simulink model "SimulacionRM20"  (R2020a)
settings: Solver=VariableStepAuto  StartTime=0.0  StopTime=inf  RelTol=1e-3
undefined symbols (not defined in the file): DiscIntNeverNeededParam, Standard_Devices, UDP_Protocol
libraries: sldrtlib x2
settings Model: Creator=alrer  LastModifiedBy=alrer

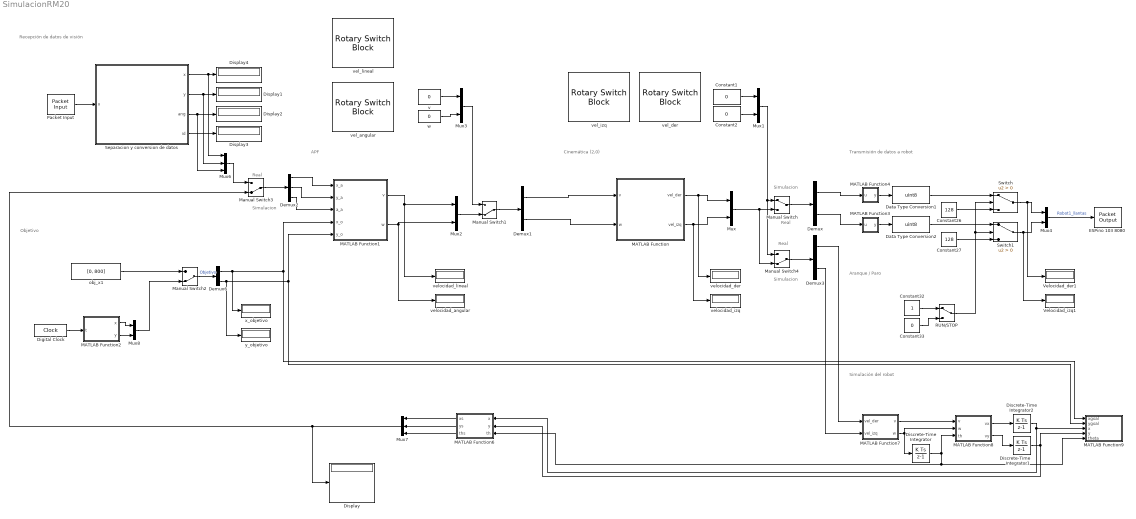
== system SimulacionRM20 ==
  note: Real
  note: Cinemática (2,0)
  note: Transmisión de datos a robot
  note: Aranque / Paro
  note: APF
  note: Objetivo
  note: Recepción de datos de visión
  note: Simulacion
  note: Simulación del robot
  note: Real
  note: Real
  note: Simulacion
  note: Simulacion
  Constant1 : Constant  Value=0
  Constant2 : Constant  Value=0
  Constant26 : Constant  Value=128
  Constant27 : Constant  Value=128
  Constant32 : Constant
  Constant33 : Constant  Value=0
  Data Type Conversion1 : DataTypeConversion  OutMin=0  OutMax=255  OutDataTypeStr=uint8
  Data Type Conversion2 : DataTypeConversion  OutMin=0  OutMax=255  OutDataTypeStr=uint8
  Demux{,1,3,6} (4 alike) : Demux  Outputs=2
  Demux2 : Demux  Outputs=3
  Digital Clock : DigitalClock  SampleTime=-1
  Discrete-Time Integrator : DiscreteIntegrator  SampleTime=-1  ICPrevOutput=DiscIntNeverNeededParam  ICPrevScaledInput=DiscIntNeverNeededParam
  Discrete-Time Integrator1 : DiscreteIntegrator  SampleTime=-1  ICPrevOutput=DiscIntNeverNeededParam  ICPrevScaledInput=DiscIntNeverNeededParam
  Discrete-Time Integrator2 : DiscreteIntegrator  SampleTime=-1  ICPrevOutput=DiscIntNeverNeededParam  ICPrevScaledInput=DiscIntNeverNeededParam
  Display{,1..4} (5 alike) : Display
  ESPino 103 8080 : sldrtlib/Packet Output  SampleTime=0.01  MaxMissedTicks=inf  ShowMissedTicks=off  YieldWhenWaiting=off  DrvName=Standard_Devices/UDP_Protocol  DrvAddress=12001  DrvOptions=[0 8080 49 57 50 46 49 54 56 46 49 51 55 46 49 55 49 0 0 0 0 0 0 0 0 0 0 0 0 0 0 0 0 0 0 0 0 0 0 0 0 0 0 0 0 0 0 0 0 0 0 0 0 0 0 0 0 0 0 0 0 0 0 0 0 0 0 0 0 0 0 0 0 0 0 0 0 0 0 0 0 0 0 0 0 0 0 0 0 0 0 0 0 0 0 0 0 0 0 0 0 0 0 0 0 0 0 0 0 0 0 0 0 0 0 0 0 0 0 0 0 0 0 0 0 0 0 0 0 0 0 0 0 0 0 0 0 0 0 0 0 0 0 0 0 0 0 0 0 0 0 0 0 0 0 0 0 0 0 0 0 0 0 0 0 0 0 0 0 0 0 0 0 0 0 0 0 0 0 0 0 0 0 0 0 0 0 0 0 0 0 0 0 0 0 0 0 0 0 0 0 0 0 0 0 0 0 0 0 0 0 0 0 0 0 0 0 0 0 0 0 0 0 0 0 0 0 0 0 0 0 0 0 0 0 0 0 0 0 0 0 0 0 0 0 0 0 0 0 0 0 0 0 0 0 0]  PacketSize=2  DataTypes='2*uint8'  ShowReady=off  ShowError=off  PacketID=1  ByteOrder=1  InitialValue=[]  FinalValue=[]
      settings: AttributesFormatString=UDP Protocol [12001]
  MATLAB Function : MATLAB Function  TreatAsAtomicUnit=on
  MATLAB Function1 : MATLAB Function  TreatAsAtomicUnit=on
  MATLAB Function2 : MATLAB Function  TreatAsAtomicUnit=on
  MATLAB Function3 : MATLAB Function  TreatAsAtomicUnit=on
  MATLAB Function4 : MATLAB Function  TreatAsAtomicUnit=on
  MATLAB Function6 : MATLAB Function  TreatAsAtomicUnit=on
  MATLAB Function7 : MATLAB Function  TreatAsAtomicUnit=on
  MATLAB Function8 : MATLAB Function  TreatAsAtomicUnit=on
  MATLAB Function9 : MATLAB Function  TreatAsAtomicUnit=on
  Manual Switch : ManualSwitch
  Manual Switch{1..4} (4 alike) : ManualSwitch  CurrentSetting=0
  Mux{,1..4,8} (6 alike) : Mux  Inputs=2
  Mux6 : Mux  Inputs=3
  Mux7 : Mux  Inputs=3
  Packet Input : sldrtlib/Packet Input  SampleTime=0.001  MaxMissedTicks=inf  ShowMissedTicks=off  YieldWhenWaiting=off  DrvName=Standard_Devices/UDP_Protocol  DrvAddress=58624  DrvOptions=[0 58624 49 50 55 46 48 46 48 46 49 0 0 0 0 0 0 0 0 0 0 0 0 0 0 0 0 0 0 0 0 0 0 0 0 0 0 0 0 0 0 0 0 0 0 0 0 0 0 0 0 0 0 0 0 0 0 0 0 0 0 0 0 0 0 0 0 0 0 0 0 0 0 0 0 0 0 0 0 0 0 0 0 0 0 0 0 0 0 0 0 0 0 0 0 0 0 0 0 0 0 0 0 0 0 0 0 0 0 0 0 0 0 0 0 0 0 0 0 0 0 0 0 0 0 0 0 0 0 0 0 0 0 0 0 0 0 0 0 0 0 0 0 0 0 0 0 0 0 0 0 0 0 0 0 0 0 0 0 0 0 0 0 0 0 0 0 0 0 0 0 0 0 0 0 0 0 0 0 0 0 0 0 0 0 0 0 0 0 0 0 0 0 0 0 0 0 0 0 0 0 0 0 0 0 0 0 0 0 0 0 0 0 0 0 0 0 0 0 0 0 0 0 0 0 0 0 0 0 0 0 0 0 0 0 0 0 0 0 0 0 0 0 0 0 0 0 0 0 0 0 0 0 0 0 0]  PacketSize=34  DataTypes='34*int8'  ShowReady=off  ShowError=off  PacketID=1  ByteOrder=1  ShowTimestamp=off
      settings: AttributesFormatString=UDP Protocol [58624]
  RUN/STOP : ManualSwitch
  Separacion y conversion de datos : MATLAB Function  TreatAsAtomicUnit=on
  Switch : Switch  Criteria=u2 > Threshold
  Switch1 : Switch  Criteria=u2 > Threshold
  "Velocidad_der1 " : Display
  Velocidad_izq1 : Display
  obj_x1 : Constant  Value=[0, 800]
  v : Constant  Value=0
  vel_angular : RotarySwitchBlock
      settings: Values={{'-100', '-50', '0', '50', '100'}, [-100 -50 0 50 100]}
  vel_der : RotarySwitchBlock
      settings: Values={{'-400', '-200', '0', '200', '400'}, [-400 -200 0 200 400]}
  vel_izq : RotarySwitchBlock
      settings: Values={{'-400', '-200', '0', '200', '400'}, [-400 -200 0 200 400]}
  vel_lineal : RotarySwitchBlock
      settings: Values={{'-20', '-10', '0', '10', '20'}, [-20000 -10000 0 10000 20000]}
  velocidad_angular : Display
  velocidad_der : Display
  velocidad_izq : Display
  velocidad_lineal : Display
  w : Constant  Value=0
  x_objetivo : Display
  y_objetivo : Display
  wires:
  Packet Input/1 -> Separacion y conversion de datos/1(u)
  Separacion y conversion de datos/1(x) -> Mux6/1, Display4/1
  Separacion y conversion de datos/2(y) -> Display1/1, Mux6/2
  Separacion y conversion de datos/3(ang) -> Display2/1, Mux6/3
  Separacion y conversion de datos/4(id) -> Display3/1
  Switch1/1 -> Velocidad_izq1/1, Mux4/2
  Constant26/1 -> Switch/3
  Switch/1 -> "Velocidad_der1 "/1, Mux4/1
  Constant27/1 -> Switch1/3
  Mux4/1 -> ESPino 103 8080/1  "Robot1_llantas"
  Constant32/1 -> RUN/STOP/1
  Constant33/1 -> RUN/STOP/2
  RUN/STOP/1 -> Switch/2, Switch1/2
  MATLAB Function1/1(v) -> velocidad_lineal/1, Mux2/1
  MATLAB Function1/2(w) -> Mux2/2, velocidad_angular/1
  Manual Switch2/1 -> Demux6/1  "Objetivo"
  Digital Clock/1 -> MATLAB Function2/1(t)
  MATLAB Function2/1(x) -> Mux8/1
  MATLAB Function2/2(y) -> Mux8/2
  Mux8/1 -> Manual Switch2/2
  Demux6/1 -> x_objetivo/1, MATLAB Function9/1(xgoal), MATLAB Function1/4(x_o)
  Demux6/2 -> y_objetivo/1, MATLAB Function9/2(ygoal), MATLAB Function1/5(y_o)
  MATLAB Function/1(vel_der) -> velocidad_der/1, Mux/1
  MATLAB Function/2(vel_izq) -> velocidad_izq/1, Mux/2
  Mux/1 -> Manual Switch4/2, Manual Switch/2
  Manual Switch/1 -> Demux/1
  Demux/2 -> MATLAB Function3/1(u)
  Demux/1 -> MATLAB Function4/1(u)
  Constant2/1 -> Mux1/2
  Constant1/1 -> Mux1/1
  Mux1/1 -> Manual Switch4/1, Manual Switch/1
  Manual Switch1/1 -> Demux1/1
  Mux2/1 -> Manual Switch1/2
  Demux1/1 -> MATLAB Function/1(v)
  Demux1/2 -> MATLAB Function/2(w)
  w/1 -> Mux3/2
  Mux3/1 -> Manual Switch1/1
  MATLAB Function3/1(y) -> Data Type Conversion2/1
  v/1 -> Mux3/1
  MATLAB Function4/1(y) -> Data Type Conversion1/1
  Data Type Conversion1/1 -> Switch/1
  Data Type Conversion2/1 -> Switch1/1
  Mux6/1 -> Manual Switch3/1
  Manual Switch3/1 -> Demux2/1
  Demux2/1 -> MATLAB Function1/1(x_a)
  Demux2/2 -> MATLAB Function1/2(y_a)
  Demux2/3 -> MATLAB Function1/3(a_a)
  MATLAB Function6/1(xs) -> Mux7/1
  Mux7/1 -> Display/1, Manual Switch3/2
  MATLAB Function7/2(w) -> Discrete-Time Integrator/1, MATLAB Function8/2(w)
  MATLAB Function7/1(v) -> MATLAB Function8/1(v)
  Discrete-Time Integrator/1 -> MATLAB Function9/5(theta), MATLAB Function6/3(th), MATLAB Function8/3(th)
  MATLAB Function8/1(vx) -> Discrete-Time Integrator2/1
  MATLAB Function8/2(vy) -> Discrete-Time Integrator1/1
  Discrete-Time Integrator2/1 -> MATLAB Function6/1(x), MATLAB Function9/3(x)
  Discrete-Time Integrator1/1 -> MATLAB Function6/2(y), MATLAB Function9/4(y)
  MATLAB Function6/2(ys) -> Mux7/2
  MATLAB Function6/3(ths) -> Mux7/3
  obj_x1/1 -> Manual Switch2/1
  Manual Switch4/1 -> Demux3/1
  Demux3/2 -> MATLAB Function7/2(vel_izq)
  Demux3/1 -> MATLAB Function7/1(vel_der)

== matlab function SimulacionRM20/MATLAB Function7 ==
  data: vel_der input; v output; vel_izq input; w output
function [v, w] = fcn(vel_der, vel_izq)

    % Parametros Robot
    r = 60;               % Radio de las llantas [mm]
    b = 85;               % Distancia del eje de desplazamiento del robot al centro de las llantas [mm]
    d = 60;               % Distancia del eje de las llantas al punto de control en la dirección de desplazamiento [mm]


    v = (r*vel_der)/2 + (r*vel_izq)/2;
    w = (r*vel_der - r*vel_izq)/(2*b);
end

== matlab function SimulacionRM20/MATLAB Function2 ==
  data: x output; t input; y output
function [x,y] = trayectoria(t)

    % Trayectoria para robot real
    %x = 300*cos(t/10)+600;
    %y = 300*sin(t/10)+450;
    
    % Trayectoria para simulacion (circunferencia)
    %x = 500*cos(30*t);
    %y = 500*sin(30*t);
    
    % Trayectoria para simulacion (lissajous)
    x = 500*sin(30*(t-pi/4));
    y = 500*cos(60*(t-pi/4) + pi/2);
    
end

== matlab function SimulacionRM20/MATLAB Function8 ==
  data: v input; vx output; w input; th input; vy output
function [vx, vy] = fcn(v, w, th)
    
    % Parametros Robot
    r = 60;               % Radio de las llantas [mm]
    b = 85;               % Distancia del eje de desplazamiento del robot al centro de las llantas [mm]
    d = 60;               % Distancia del eje de las llantas al punto de control en la dirección de desplazamiento [mm]

    vx = cos(th)*v - d*sin(th)*w;
    vy = sin(th)*v + d*cos(th)*w;

end

== matlab function SimulacionRM20/MATLAB Function9 ==
  data: xgoal input; ygoal input; x input; y input; theta input
function fcn(xgoal, ygoal, x, y, theta)
    
    % Parametros Robot
    r = 60;               % Radio de las llantas [mm]
    b = 85;               % Distancia del eje de desplazamiento del robot al centro de las llantas [mm]
    d = 60;               % Distancia del eje de las llantas al punto de control en la dirección de desplazamiento [mm]

    % Límites para la visualización de la figura
    xmin=-1000;
    xmax=1000;
    ymin=-1000;
    ymax=1000;
    
    % Dimensiones del robot
    largo_rob=160;
    ancho_rob=160;
    ancho_rueda=15;
    largo_rueda=60;
    
    hold on
    g = findobj('Marker','*');
    set(g,'Visible','off')
    plot(xgoal,ygoal,'*r','MarkerSize',6); % Marca objetivo
    plot(x,y,'.b','MarkerSize',1) % Trazar trayectoria del robot (posición)
    axis([xmin xmax ymin ymax])
    axis square
    grid on
    
    % Cuerpo
    v1=[largo_rob/2;ancho_rob/2];
    v2=[-largo_rob/2;ancho_rob/2];
    v3=[-largo_rob/2;-ancho_rob/2];
    v4=[largo_rob/2;-ancho_rob/2];
    % Llanta derecha
    v5=[-d+largo_rueda/2;b+ancho_rueda/2];
    v6=[-d-largo_rueda/2;b+ancho_rueda/2];
    v7=[-d-largo_rueda/2;b-ancho_rueda/2];
    v8=[-d+largo_rueda/2;b-ancho_rueda/2];
    % Llanta izquierda
    v9=[-d+largo_rueda/2;-b+ancho_rueda/2];
    v10=[-d-largo_rueda/2;-b+ancho_rueda/2];
    v11=[-d-largo_rueda/2;-b-ancho_rueda/2];
    v12=[-d+largo_rueda/2;-b-ancho_rueda/2];
    % Eje entre llantas
    v13=[-d;b];
    v14=[-d;-b];
    %	Rueda frontal
    v15=[60;10];
    v16=[40;10];
    v17=[40;-10];
    v18=[60;-10];

    R=[cos(theta) -sin(theta);sin(theta) cos(theta)]; % Matriz de rotación
    P=[x;y];

    v1=R*v1+P;
    v2=R*v2+P;
    v3=R*v3+P;
    v4=R*v4+P;

    v5=R*v5+P;
    v6=R*v6+P;
    v7=R*v7+P;
    v8=R*v8+P;

    v9=R*v9+P;
    v10=R*v10+P;
    v11=R*v11+P;
    v12=R*v12+P;

    v13=R*v13+P;
    v14=R*v14+P;

    v15=R*v15+P;
    v16=R*v16+P;
    v17=R*v17+P;
    v18=R*v18+P;

    rob = findobj('LineStyle','-');
    set(rob,'Visible','off')
    
    % Graficar cuerpo del robot
    mob_x=[v1(1) v2(1) v3(1) v4(1) v1(1)];
    mob_y=[v1(2) v2(2) v3(2) v4(2) v1(2)];
    plot(mob_x,mob_y,'-k','linewidth',2)

    % Graficar eje entre ruedas
    mob_x=[v13(1) v14(1)];
    mob_y=[v13(2) v14(2)];
    plot(mob_x,mob_y,'-k','linewidth',2)
    
    % Graficar rueda derecha
    mob_x=[v5(1) v6(1) v7(1) v8(1) v5(1)];
    mob_y=[v5(2) v6(2) v7(2) v8(2) v5(2)];
    plot(mob_x,mob_y,'-k','linewidth',2)

    % Graficar rueda izquierda
    mob_x=[v9(1) v10(1) v11(1) v12(1) v9(1)];
    mob_y=[v9(2) v10(2) v11(2) v12(2) v9(2)];
    plot(mob_x,mob_y,'-k','linewidth',2)

    % Graficar rueda frontal
    mob_x=[v15(1) v16(1) v17(1) v18(1) v15(1)];
    mob_y=[v15(2) v16(2) v17(2) v18(2) v15(2)];
    plot(mob_x,mob_y,'-k','linewidth',1)

    drawnow 
    hold off
    
end

== matlab function SimulacionRM20/MATLAB Function ==
  data: v input; vel_der output; w input; vel_izq output
function [vel_der, vel_izq] = fcn(v, w)
    
    %v = 100*v;
    %w = 100*w;


    % Parametros Robot
    r = 60;               % Radio de las llantas [mm]
    b = 85;               % Distancia del eje de desplazamiento del robot al centro de las llantas [mm]
    d = 60;               % Distancia del eje de las llantas al punto de control en la dirección de desplazamiento [mm]
    
    % Velocidad máxima de giro de las llantas
    %velMax = 100;         % Robot real
    velMax = 10000;         % Robot simulación
    
    % Cálculo de las velocidades de giro de las llantas
    vLlantaDer = (v + b*w)/r; % Velocidad de giro de la llanta derecha   Signo - por ajuste de los motores
    vLlantaIzq = (v - b*w)/r; % Velocidad de giro de la llanta izquierda
      
    % Límite de la velocidad máxima
    if (vLlantaDer > velMax)
        vLlantaDer = velMax;
    elseif (vLlantaDer < -velMax)
        vLlantaDer = -velMax;
    end
      
    if (vLlantaIzq > velMax)
        vLlantaIzq = velMax;
    elseif (vLlantaIzq < -velMax)
        vLlantaIzq = -velMax;
    end
    
    vel_der = vLlantaDer;
    vel_izq = vLlantaIzq;
    
%********************* Ajuste para tarjetas md25   ************************

    %vel_der = 128 + vLlantaDer;
    %vel_izq = 128 + vLlantaIzq;
    
end

== matlab function SimulacionRM20/Separacion y conversion de datos ==
  data: u input; x output; y output; ang output; id output
function [x, y, ang, id] = fcn(u)
    aux=0;
    e=zeros(17);

    for i=1:1:17
        if u(i)==77 % Identificador de inicio de cadena "M"
            aux=i;
        end
    end
    
    r=17;
    for j=1:1:r
        e(j)=u(aux+j);
    end

    id = e(16)-48;
    x=(e(2)-48)*1000+(e(3)-48)*100+(e(4)-48)*10+(e(5)-48);
    y=(e(7)-48)*1000+(e(8)-48)*100+(e(9)-48)*10+(e(10)-48);
    ang=(e(13)-48)*100 + (e(14)-48)*10 + (e(15)-48);

    if(e(1)==45)
           x = -x;
    end

    if(e(6)==45)
           y = -y;
    end
end

== matlab function SimulacionRM20/MATLAB Function1 ==
  data: x_a input; v output; y_a input; a_a input; x_o input; y_o input; w output
function [v, w] = fcn(x_a, y_a, a_a, x_o, y_o)

    % Para robot real:
    %kv = 1.5;        % Constante de proporcionalidad de velocidad lineal
    %kw = 0.1;          % Constante de proporcionalidad de velocidad angular
    %rp = 30;         % Radio de protección del robot (se considera que ya llegó al objetivo) [mm]
    %ap = 15;         % Ángulo de protección [°]
    
    % Para simulación:
    kv = 90;        % Constante de proporcionalidad de velocidad lineal
    kw = 6;          % Constante de proporcionalidad de velocidad angular
    rp = 10;         % Radio de protección del robot (se considera que ya llegó al objetivo) [mm]
    ap = 3;         % Ángulo de protección [°]

    d_obj=sqrt((x_o-x_a)^2+(y_o-y_a)^2);  %Calcula la distancia del agente al objetivo
    v = kv * d_obj;            %Velocidad hacia el objetivo es proporcional a la distancia al mismo
      
    a_o = atan2(y_o-y_a, x_o-x_a)*180/pi;    %Cálculo del ángulo con respecto al eje x del agente al objetivo
    da_obj = a_o - (a_a + 90);         %Diferencia entre ángulo del agente y ángulo al objetivo
    
    if (da_obj > 180)
        da_obj = da_obj - 360;
    end
      
    if (da_obj < -180)
        da_obj = da_obj + 360;
    end
    
    w = kw * da_obj;            %Velocidad angular es proporcional a diferencia de ángulo
    
    if (d_obj < rp)
        v = 0;
    end
    if (abs(da_obj) < ap)
        w = 0;
    end

end

== matlab function SimulacionRM20/MATLAB Function3 ==
  data: u input; y output
function y = fcn(u)

y = 128-u;

== matlab function SimulacionRM20/MATLAB Function4 ==
  data: u input; y output
function y = fcn(u)

y = 128 + u;

== matlab function SimulacionRM20/MATLAB Function6 ==
  data: x input; xs output; y input; ys output; ths output; th input
function [xs, ys, ths] = fcn(x, y, th)

    xs = x;
    ys = y;
    ths = mod((th*180/pi)-90, 360);

end
